simulink model "modeloNL"  (R2023a)
settings: Solver=FixedStepAuto  StartTime=0.0  StopTime=30  FixedStep=0.01  RelTol=1e-3
values from neighbouring files (symbols this model uses):
  CA = 8.564    [Identificacao.m]    (also in Linearizacao_CSTR.m)
  CAf = 10    [Identificacao.m]    (also in Linearizacao_CSTR.m)
  du1 = 0    [Identificacao.m]    (also in Linearizacao_CSTR.m = 0.01)
  du2 = 0    [Identificacao.m]    (also in Linearizacao_CSTR.m)
  du3 = 0    [Identificacao.m]    (also in Linearizacao_CSTR.m)
  du4 = 1    [Identificacao.m]    (also in Linearizacao_CSTR.m = 0)
  F = 1    [Identificacao.m]    (also in Linearizacao_CSTR.m)
  T = 311.2    [Identificacao.m]    (also in Linearizacao_CSTR.m; modeloDegrau.m = -Theta(3); parametrosFOPTD_igor.m = -Theta(3))
  Tf = 298    [Identificacao.m]    (also in Linearizacao_CSTR.m)
  Tj = 298    [Identificacao.m]    (also in Linearizacao_CSTR.m)
settings Model: Creator=egydi  LastModifiedBy=Mateus
settings SolverCC: AlgebraicLoopSolver=TrustRegion
settings DebuggingCC: UnconnectedInputMsg=warning  UnconnectedOutputMsg=warning  UnconnectedLineMsg=warning
settings ModelReferenceCC: EnableRefExpFcnMdlSchedulingChecks=on
settings RTWCC: DLArmComputeVersion=19.05

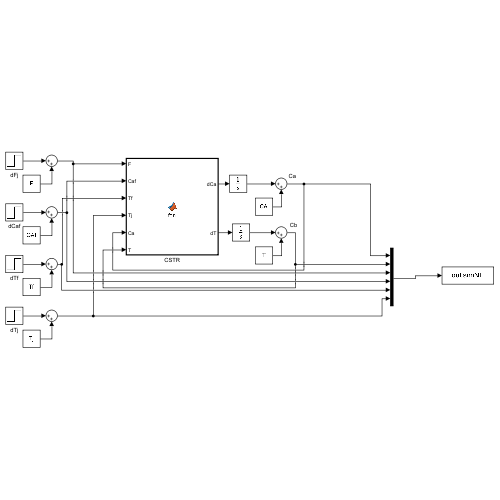
[thumbnail: Simulink's stored preview of the top-level diagram]
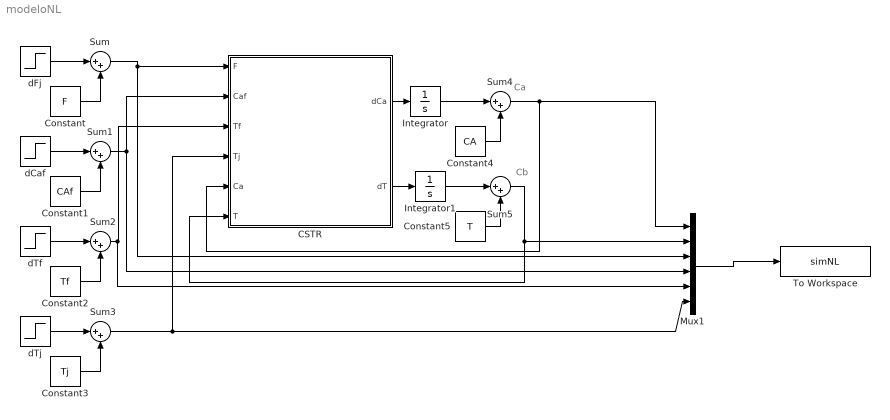
== system modeloNL ==
  note: Cb
  note: Ca
  CSTR : MATLAB Function  TreatAsAtomicUnit=on
  Constant : Constant  Value=F
  Constant1 : Constant  Value=CAf
  Constant2 : Constant  Value=Tf
  Constant3 : Constant  Value=Tj
  Constant4 : Constant  Value=CA
  Constant5 : Constant  Value=T
  Integrator : Integrator
  Integrator1 : Integrator
  Mux1 : Mux  Inputs=6
  Sum{,1..5} (6 alike) : Sum  Inputs=|++
  To Workspace : ToWorkspace  VariableName=simNL  SaveFormat=Structure With Time  SampleTime=-1
  dCaf : Step  Time=0  After=du2  SampleTime=0
  dFj : Step  Time=0  After=du1  SampleTime=0
  dTf : Step  Time=0  After=du3  SampleTime=0
  dTj : Step  Time=0  After=du4  SampleTime=0
  wires:
  CSTR/2(dT) -> Integrator1/1
  Sum5/1 -> Mux1/2, CSTR/6(T)
  Sum1/1 -> Mux1/4, CSTR/2(Caf)
  dFj/1 -> Sum/1
  Constant/1 -> Sum/2
  dCaf/1 -> Sum1/1
  Constant1/1 -> Sum1/2
  CSTR/1(dCa) -> Integrator/1
  Integrator/1 -> Sum4/1
  Integrator1/1 -> Sum5/1
  Constant4/1 -> Sum4/2
  Constant5/1 -> Sum5/2
  Mux1/1 -> To Workspace/1
  Sum/1 -> Mux1/3, CSTR/1(F)
  dTf/1 -> Sum2/1
  Constant3/1 -> Sum3/2
  Constant2/1 -> Sum2/2
  dTj/1 -> Sum3/1
  Sum2/1 -> Mux1/5, CSTR/3(Tf)
  Sum3/1 -> CSTR/4(Tj), Mux1/6
  Sum4/1 -> Mux1/1, CSTR/5(Ca)

== matlab function modeloNL/CSTR ==
  data: F input; Caf input; Tf input; Tj input; dCa output; Ca input; dT output; T input
function [dCa, dT] = fcn(F, Caf, Tf, Tj, Ca, T)

V = 1; %m^3    
dE = 11843;
rhocp = 500;
R = 1.987;

% variaveis
k0 = 9703*3600;
dH = -5960;
UA = 150;

ks = k0*exp(-dE/(R*T));

dCa = (F/V) * (Caf - Ca) - ks * Ca;
dT = (F/V) * (Tf - T) + (-dH/rhocp)*ks*Ca - (UA/(V*rhocp))*(T-Tj);
